simulink model "MJ1_2RC_EKF_v02_S2_Final"  (R2025b)
settings: Solver=FixedStepDiscrete  StartTime=0.0  StopTime=StopTime  FixedStep=1  RelTol=1e-3
undefined symbols (not defined in the file): C1_table, C2_table, OCV_table, Qref_Ah, R0_table, R1_table, R2_table, SOC0, SOC_bp, Ts, v1_0, v2_0
settings Model: Creator=louis  LastModifiedBy=louis

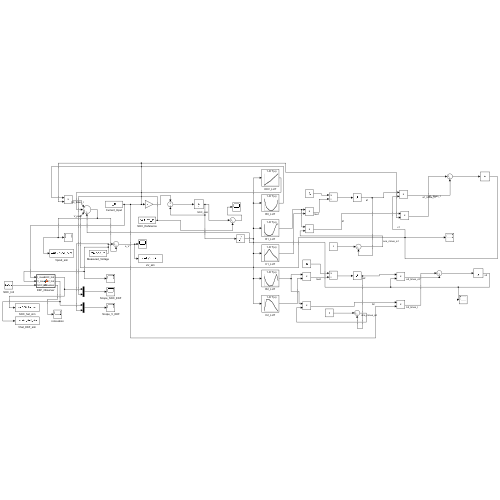
[thumbnail: Simulink's stored preview of the top-level diagram]
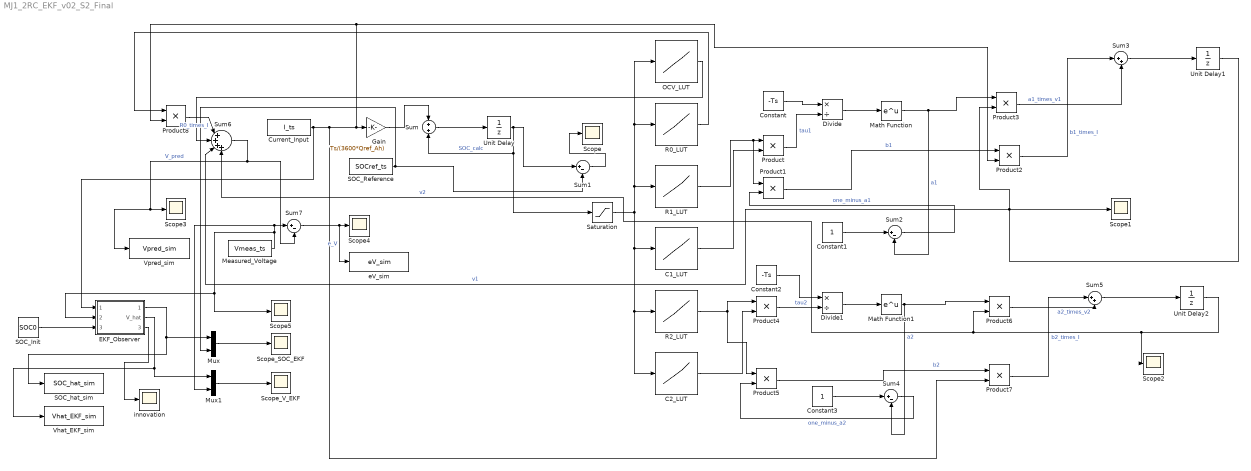
== system MJ1_2RC_EKF_v02_S2_Final ==
  " Scope_V_EKF" : Scope
      settings: DataLoggingVariableName=ScopeData7
  C1_LUT : Lookup_n-D  NumberOfTableDimensions=1  BreakpointsForDimension1=SOC_bp  Table=C1_table  InternalRulePriority=Speed  RndMeth=Simplest
  C2_LUT : Lookup_n-D  NumberOfTableDimensions=1  BreakpointsForDimension1=SOC_bp  Table=C2_table  InternalRulePriority=Speed  RndMeth=Simplest
  Constant : Constant  Value=-Ts
  Constant1 : Constant
  Constant2 : Constant  Value=-Ts
  Constant3 : Constant
  Current_Input : FromWorkspace  VariableName=I_ts  SampleTime=1  Interpolate=off  OutputAfterFinalValue=Holding final value
  Divide : Product  Inputs=*/
  Divide1 : Product  Inputs=*/
  EKF_Observer : MATLAB Function  TreatAsAtomicUnit=on
  Gain : Gain  Gain=Ts/(3600*Qref_Ah)
  Math Function : Math
  Math Function1 : Math
  Measured_Voltage : FromWorkspace  VariableName=Vmeas_ts  SampleTime=1  Interpolate=off  OutputAfterFinalValue=Holding final value
  Mux : Mux  Inputs=2
  Mux1 : Mux  Inputs=2
  OCV_LUT : Lookup_n-D  NumberOfTableDimensions=1  BreakpointsForDimension1=SOC_bp  Table=OCV_table  InternalRulePriority=Speed  RndMeth=Simplest
  Product{,1..8} (9 alike) : Product
  R0_LUT : Lookup_n-D  NumberOfTableDimensions=1  BreakpointsForDimension1=SOC_bp  Table=R0_table  InternalRulePriority=Speed  RndMeth=Simplest
  R1_LUT : Lookup_n-D  NumberOfTableDimensions=1  BreakpointsForDimension1=SOC_bp  Table=R1_table  InternalRulePriority=Speed  RndMeth=Simplest
  R2_LUT : Lookup_n-D  NumberOfTableDimensions=1  BreakpointsForDimension1=SOC_bp  Table=R2_table  InternalRulePriority=Speed  RndMeth=Simplest
  SOC_Init : Constant  Value=SOC0
  SOC_Reference : FromWorkspace  VariableName=SOCref_ts  SampleTime=1  Interpolate=off  OutputAfterFinalValue=Holding final value
  SOC_hat_sim : ToWorkspace  VariableName=SOC_hat_sim  SaveFormat=Timeseries  SampleTime=-1
  Saturation : Saturate  UpperLimit=0.85  LowerLimit=0.17
  Scope{,1..5} (6 alike) : Scope
      Scope settings: ActiveDisplayYMinimum=-0.85672073625869916  ActiveDisplayYMaximum=0.7757637466107693
      Scope1 settings: ActiveDisplayYMinimum=-1  ActiveDisplayYMaximum=1
      Scope2 settings: ActiveDisplayYMinimum=-1  ActiveDisplayYMaximum=1  DataLoggingVariableName=ScopeData2
      Scope3 settings: DataLoggingVariableName=ScopeData3
      Scope4 settings: ActiveDisplayYMinimum=-1  ActiveDisplayYMaximum=1  DataLoggingVariableName=ScopeData4
      Scope5 settings: ActiveDisplayYMinimum=-1  ActiveDisplayYMaximum=1  DataLoggingVariableName=ScopeData5
  Scope_SOC_EKF : Scope
      settings: DataLoggingVariableName=ScopeData6
  Sum : Sum
  Sum{1..2,4,7} (4 alike) : Sum  Inputs=|+-
  Sum3 : Sum  Inputs=|++
  Sum5 : Sum  Inputs=|++
  Sum6 : Sum  Inputs=|++++
  Unit Delay : UnitDelay  InitialCondition=SOC0  HasFrameUpgradeWarning=on
  Unit Delay1 : UnitDelay  InitialCondition=v1_0  HasFrameUpgradeWarning=on
  Unit Delay2 : UnitDelay  InitialCondition=v2_0  HasFrameUpgradeWarning=on
  Vhat_EKF_sim : ToWorkspace  VariableName=Vhat_EKF_sim  SaveFormat=Timeseries  SampleTime=-1
  Vpred_sim : ToWorkspace  VariableName=Vpred_sim  SaveFormat=Timeseries  SampleTime=-1
  eV_sim : ToWorkspace  VariableName=eV_sim  SaveFormat=Timeseries  SampleTime=-1
  innovation : Scope
      settings: DataLoggingVariableName=ScopeData8
  wires:
  Current_Input/1 -> EKF_Observer/1(I_meas), Product7/2, Product2/2, Product8/2, Gain/1
  Gain/1 -> Sum/1
  Sum/1 -> Unit Delay/1
  Unit Delay/1 -> Saturation/1, Sum/2, Sum1/1  "SOC_calc"
  SOC_Reference/1 -> Mux/2, Sum1/2
  Sum1/1 -> Scope/1
  Saturation/1 -> C2_LUT/1, R2_LUT/1, C1_LUT/1, R0_LUT/1, OCV_LUT/1, R1_LUT/1
  R1_LUT/1 -> Product1/1, Product/1
  C1_LUT/1 -> Product/2
  Constant/1 -> Divide/1
  Product/1 -> Divide/2  "tau1"
  Divide/1 -> Math Function/1
  Math Function/1 -> Product3/1, Sum2/2  "a1"
  Constant1/1 -> Sum2/1
  Sum2/1 -> Product1/2  "one_minus_a1"
  Product1/1 -> Product2/1  "b1"
  Unit Delay1/1 -> Product3/2, Scope1/1, Sum6/3  "v1"
  Product2/1 -> Sum3/1  "b1_times_I"
  Product3/1 -> Sum3/2  "a1_times_v1"
  Sum3/1 -> Unit Delay1/1
  R2_LUT/1 -> Product5/1, Product4/1
  C2_LUT/1 -> Product4/2
  Constant2/1 -> Divide1/1
  Product4/1 -> Divide1/2  "tau2"
  Divide1/1 -> Math Function1/1
  Sum4/1 -> Product5/2  "one_minus_a2"
  Product5/1 -> Product7/1  "b2"
  Math Function1/1 -> Sum4/2, Product6/1  "a2"
  Product6/1 -> Sum5/2  "a2_times_v2"
  Product7/1 -> Sum5/1  "b2_times_I"
  Sum5/1 -> Unit Delay2/1
  Constant3/1 -> Sum4/1
  Unit Delay2/1 -> Product6/2, Sum6/4, Scope2/1  "v2"
  R0_LUT/1 -> Product8/1
  Product8/1 -> Sum6/1  "R0_times_I"
  OCV_LUT/1 -> Sum6/2
  Sum6/1 -> Sum7/2, Vpred_sim/1, Scope3/1  "V_pred"
  Measured_Voltage/1 -> Mux1/2, Sum7/1, Scope5/1, EKF_Observer/2(V_meas)
  Sum7/1 -> eV_sim/1, Scope4/1  "e_V"
  SOC_Init/1 -> EKF_Observer/3(SOC_init)
  EKF_Observer/1(SOC_hat) -> SOC_hat_sim/1, Mux/1
  Mux/1 -> Scope_SOC_EKF/1
  EKF_Observer/2(V_hat) -> Mux1/1, Vhat_EKF_sim/1
  Mux1/1 -> " Scope_V_EKF"/1
  EKF_Observer/3(innovation) -> innovation/1

== matlab function MJ1_2RC_EKF_v02_S2_Final/EKF_Observer ==
  data: I_meas input; SOC_hat output; V_meas input; SOC_init input; V_hat output; innovation output
function [SOC_hat, V_hat, innovation] = fcn(I_meas, V_meas, SOC_init)
%#codegen
% MJ1 v0.2 SOC-dependent 2RC EKF
%
% Current sign:
%   I > 0 : charge
%   I < 0 : discharge
%
% State:
%   x = [v1; v2; SOC]

%% Frozen v0.2 model
S = coder.load('mj1_v02_model.mat','model');
model = S.model;

%% Persistent EKF states
persistent xPost PPost IPrev initialized

%% Frozen EKF settings
Q = diag([1e-7, 1e-7, 1e-9]);

sigmaV = 0.020;       % 20 mV
R = sigmaV^2;

dt = 1.0;             % 1 s sample time

%% ============================================================
% Initialization
%% ============================================================
if isempty(initialized)

    z0 = min(max(SOC_init, model.socMin), model.socMax);

    p0 = getParams(model, z0);

    % Same RC-state initialization as Python/MATLAB reference
    xPost = [ ...
        p0.R1 * I_meas; ...
        p0.R2 * I_meas; ...
        z0 ];

    PPost = diag([0.02^2, 0.02^2, 0.20^2]);

    IPrev = I_meas;

    V_hat = measurementFcn(xPost, I_meas, model);

    innovation = V_meas - V_hat;

    SOC_hat = xPost(3);

    initialized = true;
    return
end

%% ============================================================
% EKF prediction
%% ============================================================
F = processJacobian(xPost, IPrev, dt, model);

xPred = stateFcn(xPost, IPrev, dt, model);

PPred = F * PPost * F' + Q;

%% ============================================================
% Measurement prediction
%% ============================================================
V_pred = measurementFcn(xPred, I_meas, model);

innovation = V_meas - V_pred;

H = measurementJacobian(xPred, I_meas, model);

%% ============================================================
% Kalman correction
%% ============================================================
Sinnov = H * PPred * H' + R;

K = (PPred * H') / Sinnov;

xNew = xPred + K * innovation;

% Limit SOC to experimentally supported range
xNew(3) = min(max(xNew(3), model.socMin), model.socMax);

%% ============================================================
% Joseph covariance update
%% ============================================================
I3 = eye(3);

A = I3 - K * H;

PNew = A * PPred * A' + K * R * K';

% Enforce numerical symmetry
PNew = 0.5 * (PNew + PNew');

%% ============================================================
% Store posterior states
%% ============================================================
xPost = xNew;
PPost = PNew;
IPrev = I_meas;

SOC_hat = xPost(3);

V_hat = measurementFcn(xPost, I_meas, model);

end


%% ========================================================================
function xNext = stateFcn(x, currentA, dt, model)

p = getParams(model, x(3));

tau1 = p.R1 * p.C1;
tau2 = p.R2 * p.C2;

% Exact discrete RC dynamics
a1 = exp(-dt / tau1);
a2 = exp(-dt / tau2);

b1 = p.R1 * (1 - a1);
b2 = p.R2 * (1 - a2);

xNext = zeros(3,1);

xNext(1) = a1*x(1) + b1*currentA;
xNext(2) = a2*x(2) + b2*currentA;

xNext(3) = ...
    x(3) + currentA*dt/(3600*model.qRefAh);

end


%% ========================================================================
function voltageV = measurementFcn(x, currentA, model)

p = getParams(model, x(3));

voltageV = ...
    p.OCV + ...
    x(1) + ...
    x(2) + ...
    p.R0 * currentA;

end


%% ========================================================================
function F = processJacobian(x, currentA, dt, model)

epsState = [1e-6; 1e-6; 1e-5];

F = zeros(3,3);

for j = 1:3

    xp = x;
    xm = x;

    xp(j) = xp(j) + epsState(j);
    xm(j) = xm(j) - epsState(j);

    fp = stateFcn(xp, currentA, dt, model);
    fm = stateFcn(xm, currentA, dt, model);

    F(:,j) = (fp - fm) / (2*epsState(j));

end

end


%% ========================================================================
function H = measurementJacobian(x, currentA, model)

epsState = [1e-6; 1e-6; 1e-5];

H = zeros(1,3);

for j = 1:3

    xp = x;
    xm = x;

    xp(j) = xp(j) + epsState(j);
    xm(j) = xm(j) - epsState(j);

    hp = measurementFcn(xp, currentA, model);
    hm = measurementFcn(xm, currentA, model);

    H(j) = (hp - hm) / (2*epsState(j));

end

end


%% ========================================================================
function p = getParams(model, soc)

z = min(max(soc, model.socMin), model.socMax);

p.OCV = lutLinear(model.soc, model.ocv, z);

p.R0 = lutLinear(model.soc, model.R0, z);
p.R1 = lutLinear(model.soc, model.R1, z);
p.C1 = lutLinear(model.soc, model.C1, z);

p.R2 = lutLinear(model.soc, model.R2, z);
p.C2 = lutLinear(model.soc, model.C2, z);

end


%% ========================================================================
function y = lutLinear(bp, tableData, z)
% Explicit piecewise-linear interpolation

n = numel(bp);

if z <= bp(1)
    y = tableData(1);
    return
end

if z >= bp(n)
    y = tableData(n);
    return
end

y = tableData(n);

for k = 1:n-1

    if z <= bp(k+1)

        alpha = ...
            (z - bp(k)) / ...
            (bp(k+1) - bp(k));

        y = ...
            tableData(k) + ...
            alpha * (tableData(k+1) - tableData(k));

        return
    end

end

end
